simulink model "untitled3"  (R2020b)
settings: Solver=VariableStepAuto  StartTime=0.0  StopTime=10.0  RelTol=1e-3
values from neighbouring files (symbols this model uses):
  a = -3    [matlab.mat]    (also in matlab2.mat)
  b = -4    [matlab.mat]    (also in matlab2.mat)
undefined symbols (not defined in the file or in its folder): c
settings Model: Creator=sai  LastModifiedBy=sai

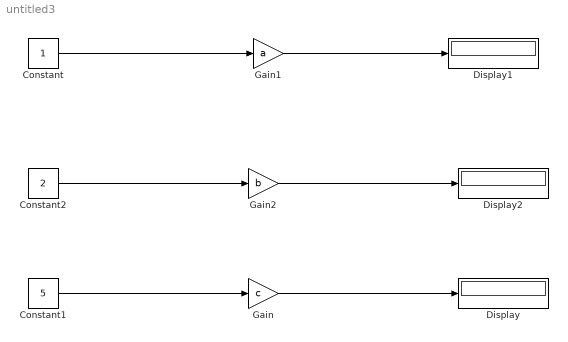
== system untitled3 ==
  Constant : Constant
  Constant1 : Constant  Value=5
  Constant2 : Constant  Value=2
  Display : Display
  Display1 : Display
  Display2 : Display
  Gain : Gain  Gain=c
  Gain1 : Gain  Gain=a
  Gain2 : Gain  Gain=b
  wires:
  Gain1/1 -> Display1/1
  Gain2/1 -> Display2/1
  Gain/1 -> Display/1
  Constant1/1 -> Gain/1
  Constant2/1 -> Gain2/1
  Constant/1 -> Gain1/1
